simulink model "dorado_tp2_simulink"  (Simulink 7.9)
settings: Solver=ode45  StartTime=0.0  StopTime=10.0  RelTol=1e-3
settings Model: Creator=diegodorado  LastModifiedBy=diegodorado

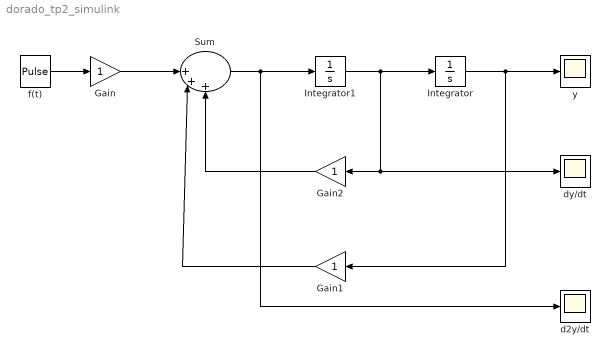
== system dorado_tp2_simulink ==
  Gain : Gain
  Gain1 : Gain
  Gain2 : Gain
  Integrator : Integrator
  Integrator1 : Integrator
  Sum : Sum  Inputs=||+++
  d2y/dt : Scope
      settings: SaveName=ScopeData2
  dy/dt : Scope
  f(t) : DiscretePulseGenerator  PulseType=Time based  Period=10  PulseWidth=5
  y : Scope
  wires:
  f(t)/1 -> Gain/1
  Gain/1 -> Sum/1
  Sum/1 -> Integrator1/1, d2y/dt/1
  Integrator1/1 -> Integrator/1, Gain2/1, dy/dt/1
  Integrator/1 -> y/1, Gain1/1
  Gain1/1 -> Sum/2
  Gain2/1 -> Sum/3
